simulink model "parallel_accumulator_test"  (Simulink 7.4)
settings: Solver=ode45  StartTime=0.0  StopTime=1000  RelTol=1e-3
undefined symbols (not defined in the file): filters_internal, Parallel_accumulator_xblock, Parallel_scope, Parallelizer, To_be_added_to_xBlocks_devels
libraries: xbsIndex_r4 x193, simulink x3
settings Model: Creator=chenhong  LastModifiedBy=chenhong

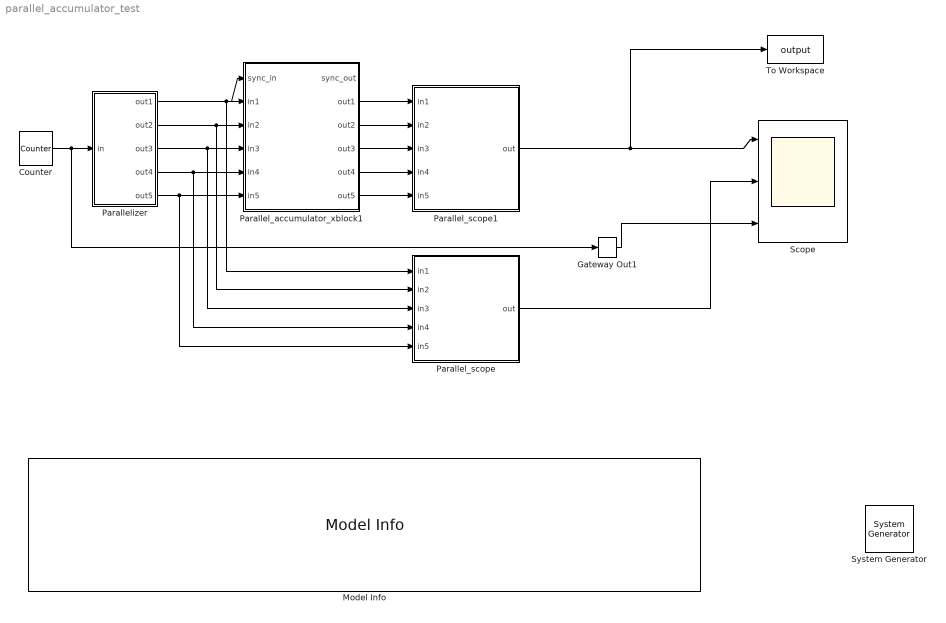
== system parallel_accumulator_test ==
  " System Generator" : xbsIndex_r4/ System Generator  Tag=genX  SystemSampleTime=-1  xilinxfamily=Virtex6  part=xc6vsx315t  speed=-3  package=ff1156  synthesis_tool=XST  clock_wrapper=Clock Enables  directory=./netlist  testbench=off  simulink_period=1  sysclk_period=10  dcm_input_clock_period=10  incr_netlist=off  trim_vbits=Everywhere in SubSystem  dbl_ovrd=According to Block Masks  core_generation=According to Block Masks  run_coregen=off  deprecated_control=off  eval_field=0  block_type=sysgen
      settings: block_version=11.4
  Counter : xbsIndex_r4/Counter  cnt_type=Free Running  cnt_to=Inf  operation=Up  start_count=0  cnt_by_val=1  arith_type=Unsigned  n_bits=8  bin_pt=0  load_pin=off  rst=off  en=off  explicit_period=on  period=1  dbl_ovrd=off  use_behavioral_HDL=off  implementation=Fabric  block_type=counter
      settings: block_version=11.4
  Gateway Out1 : xbsIndex_r4/Gateway Out  hdl_port=on  timing_constraint=None  locs_specified=off  LOCs={}  block_type=gatewayout
      settings: infoedit="Gateway out block.  Converts Xilinx fixed point inputs into ouputs of type Simulink integer, double, or fixed point.<br><br>Hardware notes:  In hardware these blocks become top level output ports or are discarded, depending on how they are configured."  block_version=11.4
  Model Info : simulink/Model-Wide Utilities/Model Info  SystemSampleTime=-1  InitialBlockCM=None  BlockCM=None  Frame=on  DisplayStringWithTags=|  HorizontalTextAlignment=Left  LeftAlignmentValue=0.02  SourceBlockDiagram=parallel_accumulator_test  TagMaxNumber=20
      | September 28, 2011:
      | 
      | Test passed. 
      | 
      | The counter generates 1-D discrete samples at 1 sample/clk rate. The parallelizer outputs 4-parallel outputs
      | at 4 sample/clk. The Parallel accumulator outputs 4-parallel outputs, each stream is the accumlated sum (for given length).
      | 
      | y(n)=x(n)+x(n-1)+x(n-2)+...+x(n-len+1)
      | 
      | Also tested: 5-parallel inputs. Various accumulation length. Various add_latency
  Parallel_accumulator_xblock1 : Subsystem  AncestorBlock=filters_internal/Parallel_accumulator_xblock  mask(Parallel Accumulator (xBlock)){n_inputs=5, len=27, add_latency=5}
      mask prompts: n_inputs "number of inputs"; len "Accumulation Lenght"; add_latency "Add Latency"
      mask help: Parallely accumulate for a given length.
      mask init:
      | config.source=str2func('parallel_accumulator_init_xblock');
      | config.depend=get_dependlist('parallel_accumulator');
      | config.toplevel=gcb;
      | set_param(gcb,'LinkStatus','inactive');
      | xBlock(config, {config.toplevel,...
      |     'n_inputs', n_inputs, ...
      |     'len', len, ...
      |     'add_latency', add_latency});
      settings: AttributesFormatString=|
      | Accumulation Length = 27
      | Add Latency = 5
      | Delay Length =1
  Parallel_scope : Subsystem  AncestorBlock=To_be_added_to_xBlocks_devels/Parallel_scope  mask(Parallel Scope){n_inputs=5, sample_period=5}
      mask prompts: n_inputs "Number of inputs"; sample_period "Sample Period"
      mask help:
      | This parallel scope can handle parallel inputs
      | by propagating though gateways and serialize into
      | one single stream. The output can then be connected
      | directly to a scope or toWorkspace.
      |
      | The sample_period desribes the parallel inputs rate.
      | For example, for a 4-inputs stream with sample_period = 1
      | (4 parallel inputs per Clk),  the output stream frequency
      | would be 4/1 = 4 (Sample/Clk)
      mask init:
      | config.source=str2func('parallel_scope_init_xblock');
      | config.depend=get_dependlist('parallel_scope');
      | config.toplevel=gcb;
      | set_param(gcb,'LinkStatus','inactive');
      | xBlock(config, {config.toplevel,...
      |     'n_inputs', n_inputs, ...
      |     'sample_period', sample_period});
      settings: AttributesFormatString=Sample Period = 5
  Parallel_scope1 : Subsystem  AncestorBlock=To_be_added_to_xBlocks_devels/Parallel_scope  mask(Parallel Scope){n_inputs=5, sample_period=5}
      mask prompts: n_inputs "Number of inputs"; sample_period "Sample Period"
      mask help:
      | This parallel scope can handle parallel inputs
      | by propagating though gateways and serialize into
      | one single stream. The output can then be connected
      | directly to a scope or toWorkspace.
      |
      | The sample_period desribes the parallel inputs rate.
      | For example, for a 4-inputs stream with sample_period = 1
      | (4 parallel inputs per Clk),  the output stream frequency
      | would be 4/1 = 4 (Sample/Clk)
      mask init: same as parallel_accumulator_test/Parallel_scope
      settings: AttributesFormatString=Sample Period = 5
  Parallelizer : Subsystem  AncestorBlock=To_be_added_to_xBlocks_devels/Parallelizer  mask(Parallelizer){n_outputs=5, sample_period=1}
      mask help:
      | Parallelizer takes in a single stream and convert it into
      | parallel outputs
      mask init:
      | config.source=str2func('parallelizer_init_xblock');
      | config.depend=get_dependlist('parallelizer');
      | config.toplevel=gcb;
      | set_param(gcb,'LinkStatus','inactive');
      | xBlock(config, {config.toplevel,...
      |     'n_outputs', n_outputs, ...
      |     'sample_period', sample_period});
      settings: AttributesFormatString=Sample Period = 1
  Scope : Scope  NumInputPorts=3
      settings: TimeRange=1000  YMin=-5~-5~-5  YMax=5~5~5
  To Workspace : ToWorkspace  VariableName=output  SampleTime=-1  SaveFormat=Structure
  wires:
  Counter/1 -> Parallelizer/1(in), Gateway Out1/1
  Parallelizer/1(out1) -> Parallel_scope/1(in1), Parallel_accumulator_xblock1/2(in1), Parallel_accumulator_xblock1/1(sync_in)
  Parallelizer/2(out2) -> Parallel_scope/2(in2), Parallel_accumulator_xblock1/3(in2)
  Parallelizer/3(out3) -> Parallel_scope/3(in3), Parallel_accumulator_xblock1/4(in3)
  Parallelizer/4(out4) -> Parallel_scope/4(in4), Parallel_accumulator_xblock1/5(in4)
  Parallel_accumulator_xblock1/2(out1) -> Parallel_scope1/1(in1)
  Parallel_accumulator_xblock1/3(out2) -> Parallel_scope1/2(in2)
  Parallel_accumulator_xblock1/4(out3) -> Parallel_scope1/3(in3)
  Parallel_accumulator_xblock1/5(out4) -> Parallel_scope1/4(in4)
  Parallel_scope1/1(out) -> Scope/1, To Workspace/1
  Parallel_scope/1(out) -> Scope/2
  Gateway Out1/1 -> Scope/3
  Parallelizer/5(out5) -> Parallel_scope/5(in5), Parallel_accumulator_xblock1/6(in5)
  Parallel_accumulator_xblock1/6(out5) -> Parallel_scope1/5(in5)

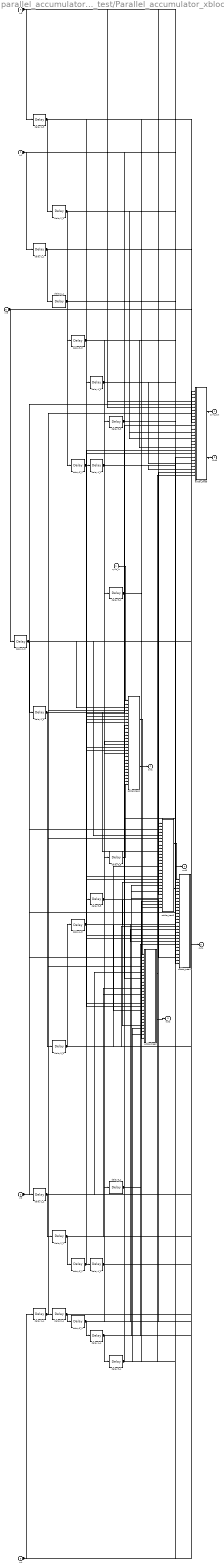
== system parallel_accumulator_test/Parallel_accumulator_xblock1 ==
  sync_in : Inport
  in1 : Inport  Port=2
  in2 : Inport  Port=3
  in3 : Inport  Port=4
  in4 : Inport  Port=5
  in5 : Inport  Port=6
  adder_tree1 : Subsystem
  adder_tree2 : Subsystem
  adder_tree3 : Subsystem
  adder_tree4 : Subsystem
  adder_tree5 : Subsystem
  delay1_{1..5} (5 alike) : xbsIndex_r4/Delay  en=off  latency=1  dbl_ovrd=off  reg_retiming=off  block_type=delay
      settings: block_version=11.4
  delay2_{1..5} (5 alike) : xbsIndex_r4/Delay  en=off  latency=1  dbl_ovrd=off  reg_retiming=off  block_type=delay
      settings: block_version=11.4
  delay3_{1..5} (5 alike) : xbsIndex_r4/Delay  en=off  latency=1  dbl_ovrd=off  reg_retiming=off  block_type=delay
      settings: block_version=11.4
  delay4_{1..5} (5 alike) : xbsIndex_r4/Delay  en=off  latency=1  dbl_ovrd=off  reg_retiming=off  block_type=delay
      settings: block_version=11.4
  delay5_{1..5} (5 alike) : xbsIndex_r4/Delay  en=off  latency=1  dbl_ovrd=off  reg_retiming=off  block_type=delay
      settings: block_version=11.4
  delay6_5 : xbsIndex_r4/Delay  en=off  latency=1  dbl_ovrd=off  reg_retiming=off  block_type=delay
      settings: block_version=11.4
  sync_out : Outport
  out1 : Outport  Port=2
  out2 : Outport  Port=3
  out3 : Outport  Port=4
  out4 : Outport  Port=5
  out5 : Outport  Port=6
  wires:
  in1/1 -> adder_tree5/6(din_5), adder_tree4/5(din_4), adder_tree3/4(din_3), adder_tree2/3(din_2), adder_tree1/2(din_1), delay1_1/1
  in2/1 -> adder_tree5/5(din_4), adder_tree4/4(din_3), adder_tree3/3(din_2), adder_tree2/2(din_1), delay1_2/1
  in3/1 -> adder_tree5/4(din_3), adder_tree4/3(din_2), adder_tree3/2(din_1), delay1_3/1
  in4/1 -> adder_tree5/3(din_2), adder_tree4/2(din_1), delay1_4/1
  in5/1 -> adder_tree5/2(din_1), delay1_5/1
  delay1_1/1 -> adder_tree5/11(din_10), adder_tree4/10(din_9), adder_tree3/9(din_8), adder_tree2/8(din_7), adder_tree1/7(din_6), delay2_1/1  "d1_1"
  delay1_2/1 -> adder_tree5/10(din_9), adder_tree4/9(din_8), adder_tree3/8(din_7), adder_tree2/7(din_6), adder_tree1/6(din_5), delay2_2/1  "d1_2"
  delay1_3/1 -> adder_tree5/9(din_8), adder_tree4/8(din_7), adder_tree3/7(din_6), adder_tree2/6(din_5), adder_tree1/5(din_4), delay2_3/1  "d1_3"
  delay1_4/1 -> adder_tree5/8(din_7), adder_tree4/7(din_6), adder_tree3/6(din_5), adder_tree2/5(din_4), adder_tree1/4(din_3), delay2_4/1  "d1_4"
  delay1_5/1 -> adder_tree5/7(din_6), adder_tree4/6(din_5), adder_tree3/5(din_4), adder_tree2/4(din_3), adder_tree1/3(din_2), delay2_5/1  "d1_5"
  delay2_1/1 -> adder_tree5/16(din_15), adder_tree4/15(din_14), adder_tree3/14(din_13), adder_tree2/13(din_12), adder_tree1/12(din_11), delay3_1/1  "d2_1"
  delay2_2/1 -> adder_tree5/15(din_14), adder_tree4/14(din_13), adder_tree3/13(din_12), adder_tree2/12(din_11), adder_tree1/11(din_10), delay3_2/1  "d2_2"
  delay2_3/1 -> adder_tree5/14(din_13), adder_tree4/13(din_12), adder_tree3/12(din_11), adder_tree2/11(din_10), adder_tree1/10(din_9), delay3_3/1  "d2_3"
  delay2_4/1 -> adder_tree5/13(din_12), adder_tree4/12(din_11), adder_tree3/11(din_10), adder_tree2/10(din_9), adder_tree1/9(din_8), delay3_4/1  "d2_4"
  delay2_5/1 -> adder_tree5/12(din_11), adder_tree4/11(din_10), adder_tree3/10(din_9), adder_tree2/9(din_8), adder_tree1/8(din_7), delay3_5/1  "d2_5"
  delay3_1/1 -> adder_tree5/21(din_20), adder_tree4/20(din_19), adder_tree3/19(din_18), adder_tree2/18(din_17), adder_tree1/17(din_16), delay4_1/1  "d3_1"
  delay3_2/1 -> adder_tree5/20(din_19), adder_tree4/19(din_18), adder_tree3/18(din_17), adder_tree2/17(din_16), adder_tree1/16(din_15), delay4_2/1  "d3_2"
  delay3_3/1 -> adder_tree5/19(din_18), adder_tree4/18(din_17), adder_tree3/17(din_16), adder_tree2/16(din_15), adder_tree1/15(din_14), delay4_3/1  "d3_3"
  delay3_4/1 -> adder_tree5/18(din_17), adder_tree4/17(din_16), adder_tree3/16(din_15), adder_tree2/15(din_14), adder_tree1/14(din_13), delay4_4/1  "d3_4"
  delay3_5/1 -> adder_tree5/17(din_16), adder_tree4/16(din_15), adder_tree3/15(din_14), adder_tree2/14(din_13), adder_tree1/13(din_12), delay4_5/1  "d3_5"
  delay4_1/1 -> adder_tree5/26(din_25), adder_tree4/25(din_24), adder_tree3/24(din_23), adder_tree2/23(din_22), adder_tree1/22(din_21), delay5_1/1  "d4_1"
  delay4_2/1 -> adder_tree5/25(din_24), adder_tree4/24(din_23), adder_tree3/23(din_22), adder_tree2/22(din_21), adder_tree1/21(din_20), delay5_2/1  "d4_2"
  delay4_3/1 -> adder_tree5/24(din_23), adder_tree4/23(din_22), adder_tree3/22(din_21), adder_tree2/21(din_20), adder_tree1/20(din_19), delay5_3/1  "d4_3"
  delay4_4/1 -> adder_tree5/23(din_22), adder_tree4/22(din_21), adder_tree3/21(din_20), adder_tree2/20(din_19), adder_tree1/19(din_18), delay5_4/1  "d4_4"
  delay4_5/1 -> adder_tree5/22(din_21), adder_tree4/21(din_20), adder_tree3/20(din_19), adder_tree2/19(din_18), adder_tree1/18(din_17), delay5_5/1  "d4_5"
  delay5_5/1 -> adder_tree5/27(din_26), adder_tree4/26(din_25), adder_tree3/25(din_24), adder_tree2/24(din_23), adder_tree1/23(din_22), delay6_5/1  "d5_5"
  delay5_4/1 -> adder_tree5/28(din_27), adder_tree4/27(din_26), adder_tree3/26(din_25), adder_tree2/25(din_24), adder_tree1/24(din_23)  "d5_4"
  delay5_3/1 -> adder_tree4/28(din_27), adder_tree3/27(din_26), adder_tree2/26(din_25), adder_tree1/25(din_24)  "d5_3"
  delay5_2/1 -> adder_tree3/28(din_27), adder_tree2/27(din_26), adder_tree1/26(din_25)  "d5_2"
  delay5_1/1 -> adder_tree2/28(din_27), adder_tree1/27(din_26)  "d5_1"
  adder_tree5/1(sync_out) -> sync_out/1  "adder_tree_sync_in5"
  adder_tree5/2(dout) -> out5/1
  adder_tree4/1(sync_out) -> adder_tree5/1(sync)  "adder_tree_sync_in4"
  adder_tree4/2(dout) -> out4/1
  adder_tree3/1(sync_out) -> adder_tree4/1(sync)  "adder_tree_sync_in3"
  adder_tree3/2(dout) -> out3/1
  adder_tree2/1(sync_out) -> adder_tree3/1(sync)  "adder_tree_sync_in2"
  adder_tree2/2(dout) -> out2/1
  adder_tree1/1(sync_out) -> adder_tree2/1(sync)  "adder_tree_sync_in1"
  adder_tree1/2(dout) -> out1/1
  delay6_5/1 -> adder_tree1/28(din_27)  "d6_5"
  sync_in/1 -> adder_tree1/1(sync)

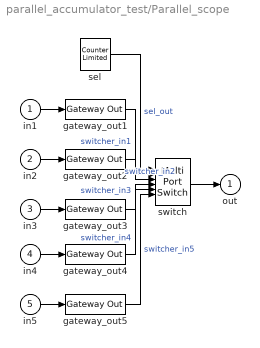
== system parallel_accumulator_test/Parallel_scope ==
  in1 : Inport
  in2 : Inport  Port=2
  in3 : Inport  Port=3
  in4 : Inport  Port=4
  in5 : Inport  Port=5
  gateway_out{1..5} (5 alike) : xbsIndex_r4/Gateway Out  hdl_port=off  timing_constraint=None  locs_specified=off  LOCs={}  block_type=gatewayout
      settings: infoedit="Gateway out block.  Converts Xilinx fixed point inputs into ouputs of type Simulink integer, double, or fixed point.<br><br>Hardware notes:  In hardware these blocks become top level output ports or are discarded, depending on how they are configured."  block_version=11.4
  sel : simulink/Sources/Counter Limited  SystemSampleTime=-1  uplimit=4  tsamp=1
  switch : MultiPortSwitch  Inputs=5  zeroidx=on  OutDataType=fixdt(1, 16)  OutScaling=2^0
  out : Outport
  wires:
  switch/1 -> out/1
  gateway_out5/1 -> switch/6  "switcher_in5"
  gateway_out4/1 -> switch/5  "switcher_in4"
  gateway_out3/1 -> switch/4  "switcher_in3"
  gateway_out2/1 -> switch/3  "switcher_in2"
  gateway_out1/1 -> switch/2  "switcher_in1"
  sel/1 -> switch/1  "sel_out"
  in5/1 -> gateway_out5/1
  in4/1 -> gateway_out4/1
  in3/1 -> gateway_out3/1
  in2/1 -> gateway_out2/1
  in1/1 -> gateway_out1/1

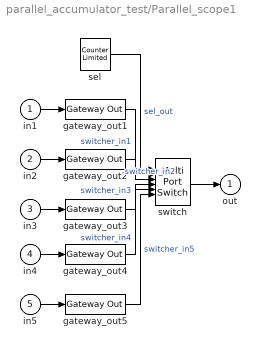
== system parallel_accumulator_test/Parallel_scope1 ==
  in1 : Inport
  in2 : Inport  Port=2
  in3 : Inport  Port=3
  in4 : Inport  Port=4
  in5 : Inport  Port=5
  gateway_out{1..5} (5 alike) : xbsIndex_r4/Gateway Out  hdl_port=off  timing_constraint=None  locs_specified=off  LOCs={}  block_type=gatewayout
      settings: infoedit="Gateway out block.  Converts Xilinx fixed point inputs into ouputs of type Simulink integer, double, or fixed point.<br><br>Hardware notes:  In hardware these blocks become top level output ports or are discarded, depending on how they are configured."  block_version=11.4
  sel : simulink/Sources/Counter Limited  SystemSampleTime=-1  uplimit=4  tsamp=1
  switch : MultiPortSwitch  Inputs=5  zeroidx=on  OutDataType=fixdt(1, 16)  OutScaling=2^0
  out : Outport
  wires:
  switch/1 -> out/1
  gateway_out5/1 -> switch/6  "switcher_in5"
  gateway_out4/1 -> switch/5  "switcher_in4"
  gateway_out3/1 -> switch/4  "switcher_in3"
  gateway_out2/1 -> switch/3  "switcher_in2"
  gateway_out1/1 -> switch/2  "switcher_in1"
  sel/1 -> switch/1  "sel_out"
  in5/1 -> gateway_out5/1
  in4/1 -> gateway_out4/1
  in3/1 -> gateway_out3/1
  in2/1 -> gateway_out2/1
  in1/1 -> gateway_out1/1

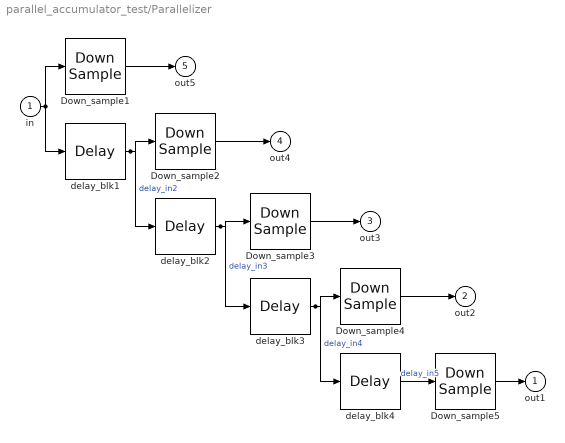
== system parallel_accumulator_test/Parallelizer ==
  in : Inport
  Down_sample{1..5} (5 alike) : xbsIndex_r4/Down Sample  sample_ratio=5  sample_phase="Last Value of Frame  (most efficient)"  en=off  latency=1  dbl_ovrd=off  block_type=dsamp
      settings: block_version=11.4
  delay_blk{1..4} (4 alike) : xbsIndex_r4/Delay  en=off  latency=1  dbl_ovrd=off  reg_retiming=off  block_type=delay
      settings: block_version=11.4
  out1 : Outport
  out2 : Outport  Port=2
  out3 : Outport  Port=3
  out4 : Outport  Port=4
  out5 : Outport  Port=5
  wires:
  in/1 -> Down_sample1/1, delay_blk1/1
  delay_blk1/1 -> Down_sample2/1, delay_blk2/1  "delay_in2"
  delay_blk2/1 -> Down_sample3/1, delay_blk3/1  "delay_in3"
  delay_blk3/1 -> Down_sample4/1, delay_blk4/1  "delay_in4"
  Down_sample5/1 -> out1/1
  delay_blk4/1 -> Down_sample5/1  "delay_in5"
  Down_sample4/1 -> out2/1
  Down_sample3/1 -> out3/1
  Down_sample2/1 -> out4/1
  Down_sample1/1 -> out5/1

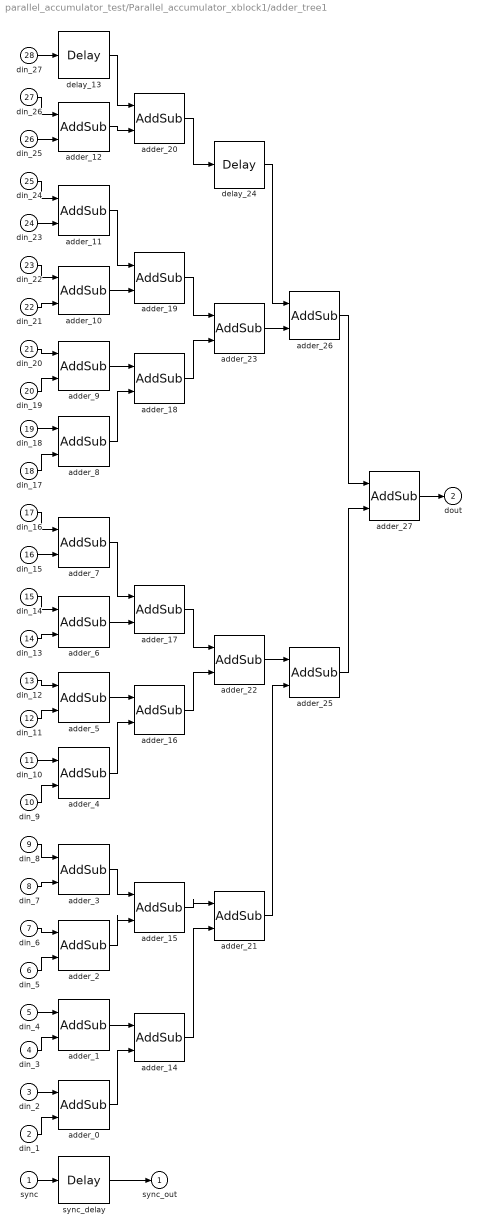
== system parallel_accumulator_test/Parallel_accumulator_xblock1/adder_tree1 ==
  sync : Inport
  din_1 : Inport  Port=2
  din_2 : Inport  Port=3
  din_3 : Inport  Port=4
  din_4 : Inport  Port=5
  din_5 : Inport  Port=6
  din_6 : Inport  Port=7
  din_7 : Inport  Port=8
  din_8 : Inport  Port=9
  din_9 : Inport  Port=10
  din_10 : Inport  Port=11
  din_11 : Inport  Port=12
  din_12 : Inport  Port=13
  din_13 : Inport  Port=14
  din_14 : Inport  Port=15
  din_15 : Inport  Port=16
  din_16 : Inport  Port=17
  din_17 : Inport  Port=18
  din_18 : Inport  Port=19
  din_19 : Inport  Port=20
  din_20 : Inport  Port=21
  din_21 : Inport  Port=22
  din_22 : Inport  Port=23
  din_23 : Inport  Port=24
  din_24 : Inport  Port=25
  din_25 : Inport  Port=26
  din_26 : Inport  Port=27
  din_27 : Inport  Port=28
  adder_{0..12,14..23,25..27} (26 alike) : xbsIndex_r4/AddSub  mode=Addition  use_carryin=off  use_carryout=off  en=off  latency=5  precision=Full  arith_type=Unsigned  n_bits=16  bin_pt=14  quantization="Round  (unbiased: +/- Inf)"  overflow=Saturate  dbl_ovrd=off  use_behavioral_HDL=on  hw_selection=Fabric  pipelined=off  block_type=addsub
  delay_13 : xbsIndex_r4/Delay  en=off  latency=5  dbl_ovrd=off  reg_retiming=off  block_type=delay
      settings: block_version=11.4
  delay_24 : xbsIndex_r4/Delay  en=off  latency=5  dbl_ovrd=off  reg_retiming=off  block_type=delay
      settings: block_version=11.4
  sync_delay : xbsIndex_r4/Delay  en=off  latency=25  dbl_ovrd=off  reg_retiming=off  block_type=delay
      settings: block_version=11.4
  sync_out : Outport
  dout : Outport  Port=2
  wires:
  adder_27/1 -> dout/1
  adder_25/1 -> adder_27/2
  adder_26/1 -> adder_27/1
  adder_23/1 -> adder_26/2
  delay_24/1 -> adder_26/1
  adder_21/1 -> adder_25/2
  adder_22/1 -> adder_25/1
  adder_20/1 -> delay_24/1
  adder_18/1 -> adder_23/2
  adder_19/1 -> adder_23/1
  adder_16/1 -> adder_22/2
  adder_17/1 -> adder_22/1
  adder_14/1 -> adder_21/2
  adder_15/1 -> adder_21/1
  adder_12/1 -> adder_20/2
  delay_13/1 -> adder_20/1
  adder_10/1 -> adder_19/2
  adder_11/1 -> adder_19/1
  adder_8/1 -> adder_18/2
  adder_9/1 -> adder_18/1
  adder_6/1 -> adder_17/2
  adder_7/1 -> adder_17/1
  adder_4/1 -> adder_16/2
  adder_5/1 -> adder_16/1
  adder_2/1 -> adder_15/2
  adder_3/1 -> adder_15/1
  adder_0/1 -> adder_14/2
  adder_1/1 -> adder_14/1
  din_27/1 -> delay_13/1
  din_25/1 -> adder_12/2
  din_26/1 -> adder_12/1
  din_23/1 -> adder_11/2
  din_24/1 -> adder_11/1
  din_21/1 -> adder_10/2
  din_22/1 -> adder_10/1
  din_19/1 -> adder_9/2
  din_20/1 -> adder_9/1
  din_17/1 -> adder_8/2
  din_18/1 -> adder_8/1
  din_15/1 -> adder_7/2
  din_16/1 -> adder_7/1
  din_13/1 -> adder_6/2
  din_14/1 -> adder_6/1
  din_11/1 -> adder_5/2
  din_12/1 -> adder_5/1
  din_9/1 -> adder_4/2
  din_10/1 -> adder_4/1
  din_7/1 -> adder_3/2
  din_8/1 -> adder_3/1
  din_5/1 -> adder_2/2
  din_6/1 -> adder_2/1
  din_3/1 -> adder_1/2
  din_4/1 -> adder_1/1
  din_1/1 -> adder_0/2
  din_2/1 -> adder_0/1
  sync_delay/1 -> sync_out/1
  sync/1 -> sync_delay/1

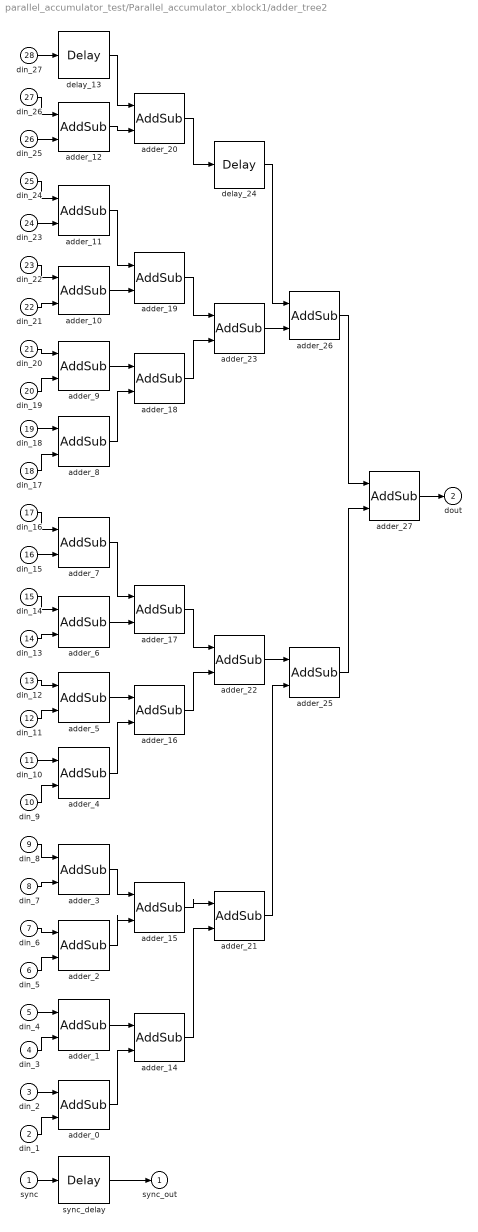
== system parallel_accumulator_test/Parallel_accumulator_xblock1/adder_tree2 ==
  sync : Inport
  din_1 : Inport  Port=2
  din_2 : Inport  Port=3
  din_3 : Inport  Port=4
  din_4 : Inport  Port=5
  din_5 : Inport  Port=6
  din_6 : Inport  Port=7
  din_7 : Inport  Port=8
  din_8 : Inport  Port=9
  din_9 : Inport  Port=10
  din_10 : Inport  Port=11
  din_11 : Inport  Port=12
  din_12 : Inport  Port=13
  din_13 : Inport  Port=14
  din_14 : Inport  Port=15
  din_15 : Inport  Port=16
  din_16 : Inport  Port=17
  din_17 : Inport  Port=18
  din_18 : Inport  Port=19
  din_19 : Inport  Port=20
  din_20 : Inport  Port=21
  din_21 : Inport  Port=22
  din_22 : Inport  Port=23
  din_23 : Inport  Port=24
  din_24 : Inport  Port=25
  din_25 : Inport  Port=26
  din_26 : Inport  Port=27
  din_27 : Inport  Port=28
  adder_{0..12,14..23,25..27} (26 alike) : xbsIndex_r4/AddSub  mode=Addition  use_carryin=off  use_carryout=off  en=off  latency=5  precision=Full  arith_type=Unsigned  n_bits=16  bin_pt=14  quantization="Round  (unbiased: +/- Inf)"  overflow=Saturate  dbl_ovrd=off  use_behavioral_HDL=on  hw_selection=Fabric  pipelined=off  block_type=addsub
  delay_13 : xbsIndex_r4/Delay  en=off  latency=5  dbl_ovrd=off  reg_retiming=off  block_type=delay
      settings: block_version=11.4
  delay_24 : xbsIndex_r4/Delay  en=off  latency=5  dbl_ovrd=off  reg_retiming=off  block_type=delay
      settings: block_version=11.4
  sync_delay : xbsIndex_r4/Delay  en=off  latency=25  dbl_ovrd=off  reg_retiming=off  block_type=delay
      settings: block_version=11.4
  sync_out : Outport
  dout : Outport  Port=2
  wires:
  adder_27/1 -> dout/1
  adder_25/1 -> adder_27/2
  adder_26/1 -> adder_27/1
  adder_23/1 -> adder_26/2
  delay_24/1 -> adder_26/1
  adder_21/1 -> adder_25/2
  adder_22/1 -> adder_25/1
  adder_20/1 -> delay_24/1
  adder_18/1 -> adder_23/2
  adder_19/1 -> adder_23/1
  adder_16/1 -> adder_22/2
  adder_17/1 -> adder_22/1
  adder_14/1 -> adder_21/2
  adder_15/1 -> adder_21/1
  adder_12/1 -> adder_20/2
  delay_13/1 -> adder_20/1
  adder_10/1 -> adder_19/2
  adder_11/1 -> adder_19/1
  adder_8/1 -> adder_18/2
  adder_9/1 -> adder_18/1
  adder_6/1 -> adder_17/2
  adder_7/1 -> adder_17/1
  adder_4/1 -> adder_16/2
  adder_5/1 -> adder_16/1
  adder_2/1 -> adder_15/2
  adder_3/1 -> adder_15/1
  adder_0/1 -> adder_14/2
  adder_1/1 -> adder_14/1
  din_27/1 -> delay_13/1
  din_25/1 -> adder_12/2
  din_26/1 -> adder_12/1
  din_23/1 -> adder_11/2
  din_24/1 -> adder_11/1
  din_21/1 -> adder_10/2
  din_22/1 -> adder_10/1
  din_19/1 -> adder_9/2
  din_20/1 -> adder_9/1
  din_17/1 -> adder_8/2
  din_18/1 -> adder_8/1
  din_15/1 -> adder_7/2
  din_16/1 -> adder_7/1
  din_13/1 -> adder_6/2
  din_14/1 -> adder_6/1
  din_11/1 -> adder_5/2
  din_12/1 -> adder_5/1
  din_9/1 -> adder_4/2
  din_10/1 -> adder_4/1
  din_7/1 -> adder_3/2
  din_8/1 -> adder_3/1
  din_5/1 -> adder_2/2
  din_6/1 -> adder_2/1
  din_3/1 -> adder_1/2
  din_4/1 -> adder_1/1
  din_1/1 -> adder_0/2
  din_2/1 -> adder_0/1
  sync_delay/1 -> sync_out/1
  sync/1 -> sync_delay/1

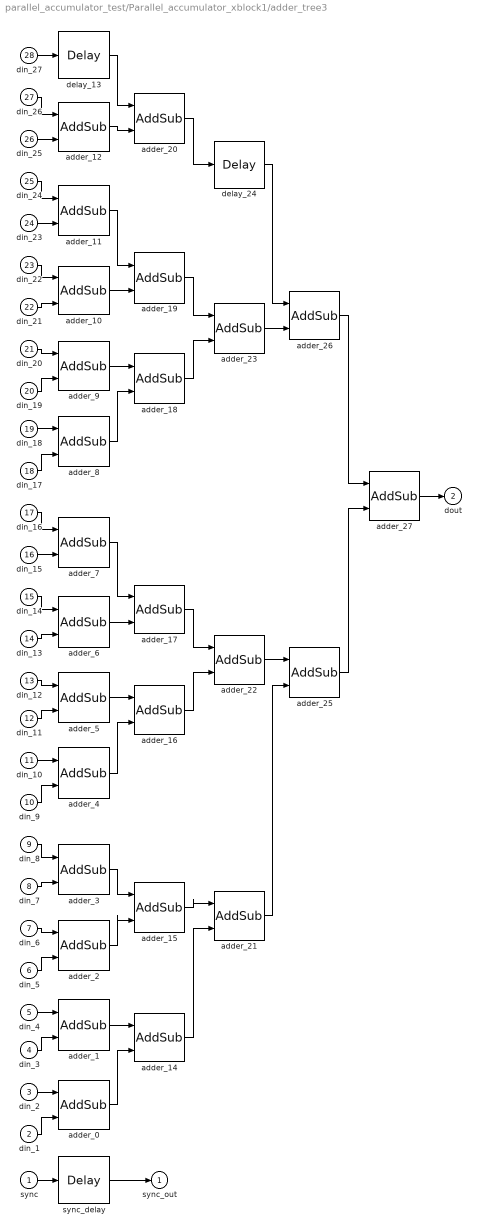
== system parallel_accumulator_test/Parallel_accumulator_xblock1/adder_tree3 ==
  sync : Inport
  din_1 : Inport  Port=2
  din_2 : Inport  Port=3
  din_3 : Inport  Port=4
  din_4 : Inport  Port=5
  din_5 : Inport  Port=6
  din_6 : Inport  Port=7
  din_7 : Inport  Port=8
  din_8 : Inport  Port=9
  din_9 : Inport  Port=10
  din_10 : Inport  Port=11
  din_11 : Inport  Port=12
  din_12 : Inport  Port=13
  din_13 : Inport  Port=14
  din_14 : Inport  Port=15
  din_15 : Inport  Port=16
  din_16 : Inport  Port=17
  din_17 : Inport  Port=18
  din_18 : Inport  Port=19
  din_19 : Inport  Port=20
  din_20 : Inport  Port=21
  din_21 : Inport  Port=22
  din_22 : Inport  Port=23
  din_23 : Inport  Port=24
  din_24 : Inport  Port=25
  din_25 : Inport  Port=26
  din_26 : Inport  Port=27
  din_27 : Inport  Port=28
  adder_{0..12,14..23,25..27} (26 alike) : xbsIndex_r4/AddSub  mode=Addition  use_carryin=off  use_carryout=off  en=off  latency=5  precision=Full  arith_type=Unsigned  n_bits=16  bin_pt=14  quantization="Round  (unbiased: +/- Inf)"  overflow=Saturate  dbl_ovrd=off  use_behavioral_HDL=on  hw_selection=Fabric  pipelined=off  block_type=addsub
  delay_13 : xbsIndex_r4/Delay  en=off  latency=5  dbl_ovrd=off  reg_retiming=off  block_type=delay
      settings: block_version=11.4
  delay_24 : xbsIndex_r4/Delay  en=off  latency=5  dbl_ovrd=off  reg_retiming=off  block_type=delay
      settings: block_version=11.4
  sync_delay : xbsIndex_r4/Delay  en=off  latency=25  dbl_ovrd=off  reg_retiming=off  block_type=delay
      settings: block_version=11.4
  sync_out : Outport
  dout : Outport  Port=2
  wires:
  adder_27/1 -> dout/1
  adder_25/1 -> adder_27/2
  adder_26/1 -> adder_27/1
  adder_23/1 -> adder_26/2
  delay_24/1 -> adder_26/1
  adder_21/1 -> adder_25/2
  adder_22/1 -> adder_25/1
  adder_20/1 -> delay_24/1
  adder_18/1 -> adder_23/2
  adder_19/1 -> adder_23/1
  adder_16/1 -> adder_22/2
  adder_17/1 -> adder_22/1
  adder_14/1 -> adder_21/2
  adder_15/1 -> adder_21/1
  adder_12/1 -> adder_20/2
  delay_13/1 -> adder_20/1
  adder_10/1 -> adder_19/2
  adder_11/1 -> adder_19/1
  adder_8/1 -> adder_18/2
  adder_9/1 -> adder_18/1
  adder_6/1 -> adder_17/2
  adder_7/1 -> adder_17/1
  adder_4/1 -> adder_16/2
  adder_5/1 -> adder_16/1
  adder_2/1 -> adder_15/2
  adder_3/1 -> adder_15/1
  adder_0/1 -> adder_14/2
  adder_1/1 -> adder_14/1
  din_27/1 -> delay_13/1
  din_25/1 -> adder_12/2
  din_26/1 -> adder_12/1
  din_23/1 -> adder_11/2
  din_24/1 -> adder_11/1
  din_21/1 -> adder_10/2
  din_22/1 -> adder_10/1
  din_19/1 -> adder_9/2
  din_20/1 -> adder_9/1
  din_17/1 -> adder_8/2
  din_18/1 -> adder_8/1
  din_15/1 -> adder_7/2
  din_16/1 -> adder_7/1
  din_13/1 -> adder_6/2
  din_14/1 -> adder_6/1
  din_11/1 -> adder_5/2
  din_12/1 -> adder_5/1
  din_9/1 -> adder_4/2
  din_10/1 -> adder_4/1
  din_7/1 -> adder_3/2
  din_8/1 -> adder_3/1
  din_5/1 -> adder_2/2
  din_6/1 -> adder_2/1
  din_3/1 -> adder_1/2
  din_4/1 -> adder_1/1
  din_1/1 -> adder_0/2
  din_2/1 -> adder_0/1
  sync_delay/1 -> sync_out/1
  sync/1 -> sync_delay/1

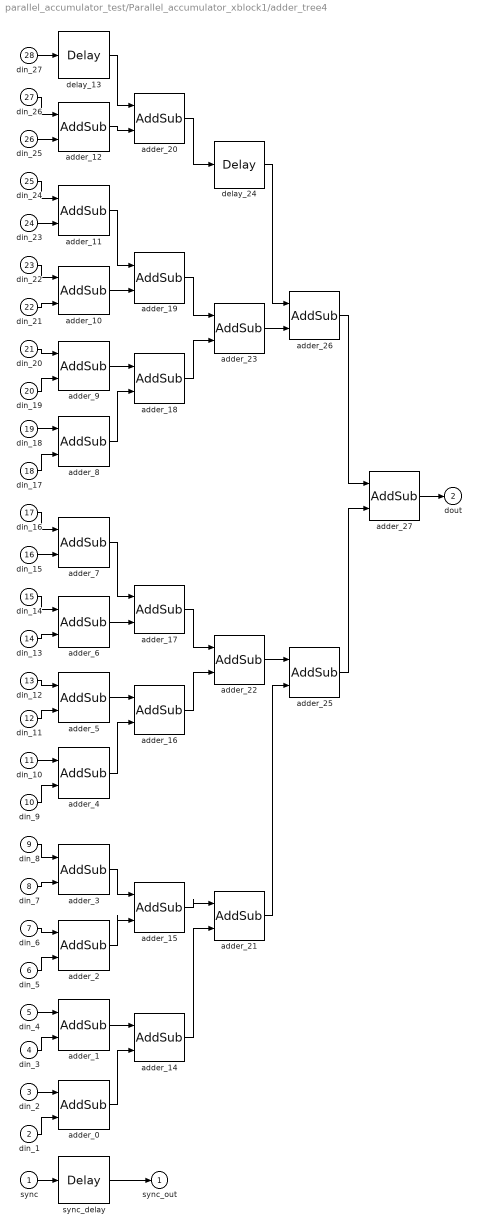
== system parallel_accumulator_test/Parallel_accumulator_xblock1/adder_tree4 ==
  sync : Inport
  din_1 : Inport  Port=2
  din_2 : Inport  Port=3
  din_3 : Inport  Port=4
  din_4 : Inport  Port=5
  din_5 : Inport  Port=6
  din_6 : Inport  Port=7
  din_7 : Inport  Port=8
  din_8 : Inport  Port=9
  din_9 : Inport  Port=10
  din_10 : Inport  Port=11
  din_11 : Inport  Port=12
  din_12 : Inport  Port=13
  din_13 : Inport  Port=14
  din_14 : Inport  Port=15
  din_15 : Inport  Port=16
  din_16 : Inport  Port=17
  din_17 : Inport  Port=18
  din_18 : Inport  Port=19
  din_19 : Inport  Port=20
  din_20 : Inport  Port=21
  din_21 : Inport  Port=22
  din_22 : Inport  Port=23
  din_23 : Inport  Port=24
  din_24 : Inport  Port=25
  din_25 : Inport  Port=26
  din_26 : Inport  Port=27
  din_27 : Inport  Port=28
  adder_{0..12,14..23,25..27} (26 alike) : xbsIndex_r4/AddSub  mode=Addition  use_carryin=off  use_carryout=off  en=off  latency=5  precision=Full  arith_type=Unsigned  n_bits=16  bin_pt=14  quantization="Round  (unbiased: +/- Inf)"  overflow=Saturate  dbl_ovrd=off  use_behavioral_HDL=on  hw_selection=Fabric  pipelined=off  block_type=addsub
  delay_13 : xbsIndex_r4/Delay  en=off  latency=5  dbl_ovrd=off  reg_retiming=off  block_type=delay
      settings: block_version=11.4
  delay_24 : xbsIndex_r4/Delay  en=off  latency=5  dbl_ovrd=off  reg_retiming=off  block_type=delay
      settings: block_version=11.4
  sync_delay : xbsIndex_r4/Delay  en=off  latency=25  dbl_ovrd=off  reg_retiming=off  block_type=delay
      settings: block_version=11.4
  sync_out : Outport
  dout : Outport  Port=2
  wires:
  adder_27/1 -> dout/1
  adder_25/1 -> adder_27/2
  adder_26/1 -> adder_27/1
  adder_23/1 -> adder_26/2
  delay_24/1 -> adder_26/1
  adder_21/1 -> adder_25/2
  adder_22/1 -> adder_25/1
  adder_20/1 -> delay_24/1
  adder_18/1 -> adder_23/2
  adder_19/1 -> adder_23/1
  adder_16/1 -> adder_22/2
  adder_17/1 -> adder_22/1
  adder_14/1 -> adder_21/2
  adder_15/1 -> adder_21/1
  adder_12/1 -> adder_20/2
  delay_13/1 -> adder_20/1
  adder_10/1 -> adder_19/2
  adder_11/1 -> adder_19/1
  adder_8/1 -> adder_18/2
  adder_9/1 -> adder_18/1
  adder_6/1 -> adder_17/2
  adder_7/1 -> adder_17/1
  adder_4/1 -> adder_16/2
  adder_5/1 -> adder_16/1
  adder_2/1 -> adder_15/2
  adder_3/1 -> adder_15/1
  adder_0/1 -> adder_14/2
  adder_1/1 -> adder_14/1
  din_27/1 -> delay_13/1
  din_25/1 -> adder_12/2
  din_26/1 -> adder_12/1
  din_23/1 -> adder_11/2
  din_24/1 -> adder_11/1
  din_21/1 -> adder_10/2
  din_22/1 -> adder_10/1
  din_19/1 -> adder_9/2
  din_20/1 -> adder_9/1
  din_17/1 -> adder_8/2
  din_18/1 -> adder_8/1
  din_15/1 -> adder_7/2
  din_16/1 -> adder_7/1
  din_13/1 -> adder_6/2
  din_14/1 -> adder_6/1
  din_11/1 -> adder_5/2
  din_12/1 -> adder_5/1
  din_9/1 -> adder_4/2
  din_10/1 -> adder_4/1
  din_7/1 -> adder_3/2
  din_8/1 -> adder_3/1
  din_5/1 -> adder_2/2
  din_6/1 -> adder_2/1
  din_3/1 -> adder_1/2
  din_4/1 -> adder_1/1
  din_1/1 -> adder_0/2
  din_2/1 -> adder_0/1
  sync_delay/1 -> sync_out/1
  sync/1 -> sync_delay/1

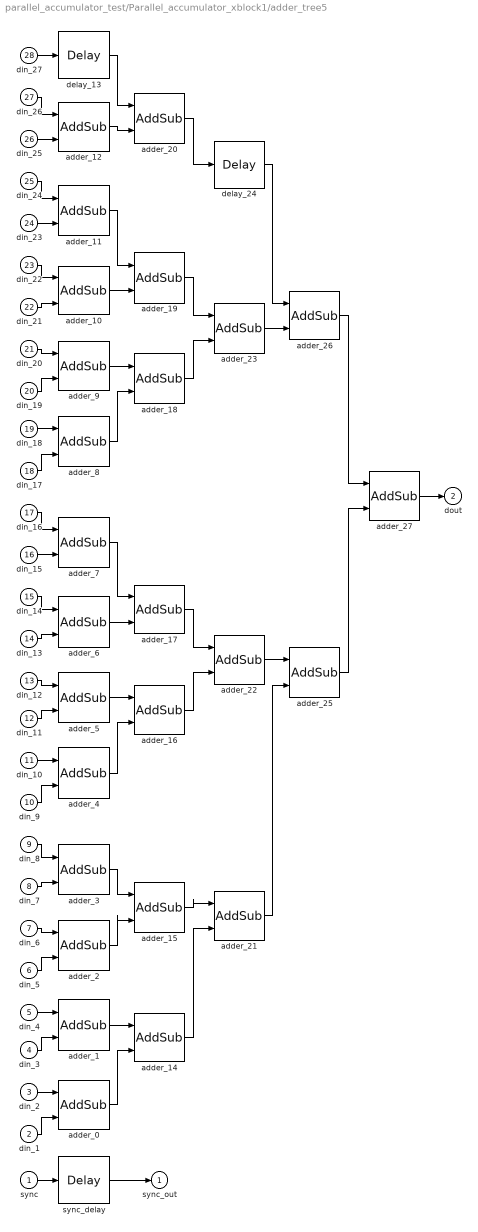
== system parallel_accumulator_test/Parallel_accumulator_xblock1/adder_tree5 ==
  sync : Inport
  din_1 : Inport  Port=2
  din_2 : Inport  Port=3
  din_3 : Inport  Port=4
  din_4 : Inport  Port=5
  din_5 : Inport  Port=6
  din_6 : Inport  Port=7
  din_7 : Inport  Port=8
  din_8 : Inport  Port=9
  din_9 : Inport  Port=10
  din_10 : Inport  Port=11
  din_11 : Inport  Port=12
  din_12 : Inport  Port=13
  din_13 : Inport  Port=14
  din_14 : Inport  Port=15
  din_15 : Inport  Port=16
  din_16 : Inport  Port=17
  din_17 : Inport  Port=18
  din_18 : Inport  Port=19
  din_19 : Inport  Port=20
  din_20 : Inport  Port=21
  din_21 : Inport  Port=22
  din_22 : Inport  Port=23
  din_23 : Inport  Port=24
  din_24 : Inport  Port=25
  din_25 : Inport  Port=26
  din_26 : Inport  Port=27
  din_27 : Inport  Port=28
  adder_{0..12,14..23,25..27} (26 alike) : xbsIndex_r4/AddSub  mode=Addition  use_carryin=off  use_carryout=off  en=off  latency=5  precision=Full  arith_type=Unsigned  n_bits=16  bin_pt=14  quantization="Round  (unbiased: +/- Inf)"  overflow=Saturate  dbl_ovrd=off  use_behavioral_HDL=on  hw_selection=Fabric  pipelined=off  block_type=addsub
  delay_13 : xbsIndex_r4/Delay  en=off  latency=5  dbl_ovrd=off  reg_retiming=off  block_type=delay
      settings: block_version=11.4
  delay_24 : xbsIndex_r4/Delay  en=off  latency=5  dbl_ovrd=off  reg_retiming=off  block_type=delay
      settings: block_version=11.4
  sync_delay : xbsIndex_r4/Delay  en=off  latency=25  dbl_ovrd=off  reg_retiming=off  block_type=delay
      settings: block_version=11.4
  sync_out : Outport
  dout : Outport  Port=2
  wires:
  adder_27/1 -> dout/1
  adder_25/1 -> adder_27/2
  adder_26/1 -> adder_27/1
  adder_23/1 -> adder_26/2
  delay_24/1 -> adder_26/1
  adder_21/1 -> adder_25/2
  adder_22/1 -> adder_25/1
  adder_20/1 -> delay_24/1
  adder_18/1 -> adder_23/2
  adder_19/1 -> adder_23/1
  adder_16/1 -> adder_22/2
  adder_17/1 -> adder_22/1
  adder_14/1 -> adder_21/2
  adder_15/1 -> adder_21/1
  adder_12/1 -> adder_20/2
  delay_13/1 -> adder_20/1
  adder_10/1 -> adder_19/2
  adder_11/1 -> adder_19/1
  adder_8/1 -> adder_18/2
  adder_9/1 -> adder_18/1
  adder_6/1 -> adder_17/2
  adder_7/1 -> adder_17/1
  adder_4/1 -> adder_16/2
  adder_5/1 -> adder_16/1
  adder_2/1 -> adder_15/2
  adder_3/1 -> adder_15/1
  adder_0/1 -> adder_14/2
  adder_1/1 -> adder_14/1
  din_27/1 -> delay_13/1
  din_25/1 -> adder_12/2
  din_26/1 -> adder_12/1
  din_23/1 -> adder_11/2
  din_24/1 -> adder_11/1
  din_21/1 -> adder_10/2
  din_22/1 -> adder_10/1
  din_19/1 -> adder_9/2
  din_20/1 -> adder_9/1
  din_17/1 -> adder_8/2
  din_18/1 -> adder_8/1
  din_15/1 -> adder_7/2
  din_16/1 -> adder_7/1
  din_13/1 -> adder_6/2
  din_14/1 -> adder_6/1
  din_11/1 -> adder_5/2
  din_12/1 -> adder_5/1
  din_9/1 -> adder_4/2
  din_10/1 -> adder_4/1
  din_7/1 -> adder_3/2
  din_8/1 -> adder_3/1
  din_5/1 -> adder_2/2
  din_6/1 -> adder_2/1
  din_3/1 -> adder_1/2
  din_4/1 -> adder_1/1
  din_1/1 -> adder_0/2
  din_2/1 -> adder_0/1
  sync_delay/1 -> sync_out/1
  sync/1 -> sync_delay/1
